simulink model "exp02"  (R2018b)
settings: Solver=VariableStepAuto  StartTime=0.0  StopTime=10.0  RelTol=1e-3
values from neighbouring files (symbols this model uses):
  B = 4    [exp02.m]
  F = 8    [exp02.m]
  K = 16    [exp02.m]
  M = 2    [exp02.m]
settings Model: Creator=student  LastModifiedBy=student

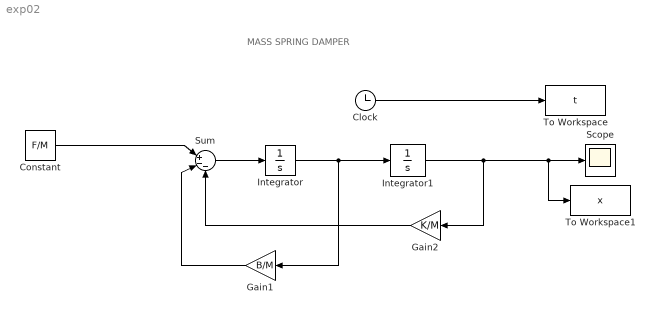
== system exp02 ==
  note: MASS SPRING DAMPER
  Clock : Clock
  Constant : Constant  Value=F/M
  Gain1 : Gain  Gain=B/M
  Gain2 : Gain  Gain=K/M
  Integrator : Integrator
  Integrator1 : Integrator  InitialCondition=5
  Scope : Scope
  Sum : Sum  Inputs=|+--
  To Workspace : ToWorkspace  VariableName=t  SampleTime=-1
  To Workspace1 : ToWorkspace  VariableName=x  SampleTime=-1
  wires:
  Gain1/1 -> Sum/2
  Sum/1 -> Integrator/1
  Gain2/1 -> Sum/3
  Integrator1/1 -> Gain2/1, To Workspace1/1, Scope/1
  Integrator/1 -> Gain1/1, Integrator1/1
  Clock/1 -> To Workspace/1
  Constant/1 -> Sum/1
